simulink model "Beclhoff_Matlab_SimulinkPositionControl"  (R2019a)
settings: Solver=ode3  StartTime=0.0  StopTime=10.0  RelTol=1e-3
libraries: TcTargetLib x7, simulink x1
settings Model: Creator=ChrisK  LastModifiedBy=cknig
settings OptimizationCC: LocalBlockOutputs=off
settings RTWCC: SystemTargetFile=TwinCAT.tlc  GenCodeOnly=on  MakeCommand=make_tct  TemplateMakefile=tct_msbuild.tmf  Description=TwinCAT Target  GenerateReport=on  TargetLang=C++
settings STFCustomTargetCC: TargetLangStandard=C++03 (ISO)  CompOptLevelCompliant=on  MATLABClassNameForMDSCustomization=Simulink.SoftwareTarget.TargetSpecificTriggerConfigurationBase  SystemTargetFile=TwinCAT.tlc

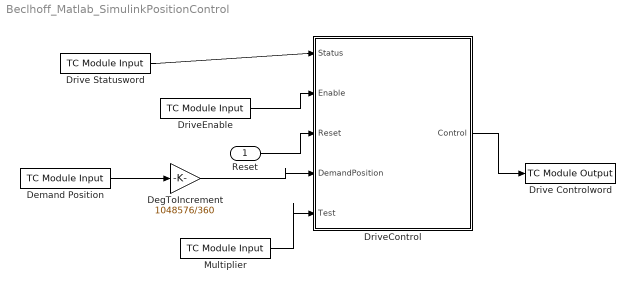
== system Beclhoff_Matlab_SimulinkPositionControl ==
  Reset : Inport  OutDataTypeStr=boolean
  DegToIncrement : Gain  Gain=1048576/360  OutDataTypeStr=int32
  Demand Position : TcTargetLib/TC Module Input  PortDataType=uint8  PortDim=1  Value=0  SampleTime=-1  CodeGenConnectType=DataArea (InputDst)
      settings: SourceProductName=Beckhoff TwinCAT Target
  "Drive Controlword " : TcTargetLib/TC Module Output  PortDataType=uint16  PortDim=1  SampleTime=-1  CodeGenConnectType=DataArea (OutputSrc)
      settings: SourceProductName=Beckhoff TwinCAT Target
  "Drive Statusword " : TcTargetLib/TC Module Input  PortDataType=uint8  PortDim=1  Value=0  SampleTime=-1  CodeGenConnectType=DataArea (InputDst)
      settings: SourceProductName=Beckhoff TwinCAT Target
  DriveControl : Stateflow chart  BlockKeywords=__PRM__SERIALIZED__DATA__:Stateflow Chart,Stateflow Diagram  TreatAsAtomicUnit=on
  DriveEnable : TcTargetLib/TC Module Input  PortDataType=boolean  PortDim=1  Value=0  SampleTime=-1  CodeGenConnectType=DataArea (InputDst)
      settings: SourceProductName=Beckhoff TwinCAT Target
  "Multiplier " : TcTargetLib/TC Module Input  PortDataType=int32  PortDim=1  Value=0  SampleTime=-1  CodeGenConnectType=DataArea (InputDst)
      settings: SourceProductName=Beckhoff TwinCAT Target
  wires:
  "Drive Statusword "/1 -> DriveControl/1(Status)
  DriveControl/1(Control) -> "Drive Controlword "/1
  DriveEnable/1 -> DriveControl/2(Enable)
  Reset/1 -> DriveControl/3(Reset)
  Demand Position/1 -> DegToIncrement/1
  DegToIncrement/1 -> DriveControl/4(DemandPosition)
  "Multiplier "/1 -> DriveControl/5(Test)

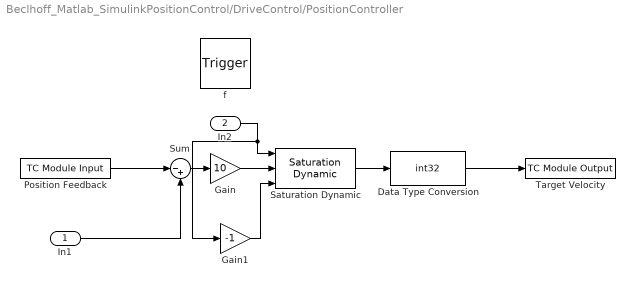
== system Beclhoff_Matlab_SimulinkPositionControl/DriveControl/PositionController ==
  In1 : Inport  OutDataTypeStr=int32  PortDimensions=1
  In2 : Inport  Port=2  OutDataTypeStr=int32  PortDimensions=1
  f : TriggerPort  TriggerType=function-call  VariantControl=(inherit)
      settings: CopyFcn=Stateflow.SLINSF.SimulinkMan.removeBlockPreDeleteFcn  PreDeleteFcn=Stateflow.SLINSF.SimulinkMan.unsafePredeleteFcn
  Data Type Conversion : DataTypeConversion  OutDataTypeStr=int32  SaturateOnIntegerOverflow=on
  Gain : Gain  Gain=10
  Gain1 : Gain  Gain=-1
  "Position Feedback " : TcTargetLib/TC Module Input  PortDataType=int32  PortDim=1  Value=0  SampleTime=-1  CodeGenConnectType=DataArea (InputDst)
      settings: SourceProductName=Beckhoff TwinCAT Target
  Saturation Dynamic : simulink/Discontinuities/Saturation Dynamic  OutMin=[]  OutMax=[]  OutDataTypeStr=Inherit: Same as second input  OutDataType=fixdt(1, 16)  OutScaling=2^-10  DoSatur=off
  Sum : Sum  Inputs=|-+
  Target Velocity : TcTargetLib/TC Module Output  PortDataType=int32  PortDim=1  SampleTime=-1  CodeGenConnectType=DataArea (OutputSrc)
      settings: SourceProductName=Beckhoff TwinCAT Target
  wires:
  Sum/1 -> Gain/1
  "Position Feedback "/1 -> Sum/1
  Data Type Conversion/1 -> Target Velocity/1
  In1/1 -> Sum/2
  Saturation Dynamic/1 -> Data Type Conversion/1
  Gain/1 -> Saturation Dynamic/2
  In2/1 -> Gain1/1, Saturation Dynamic/1
  Gain1/1 -> Saturation Dynamic/3

== stateflow chart Beclhoff_Matlab_SimulinkPositionControl/DriveControl ==
  state NotReady
    entry: Control = 128;
  state SwitchOnDisabled
    entry: Control = 6;
  state WaitForSafety
  state Resetting
    entry: Control = 128;
  state ReadyToSwitchOn
    entry: Control = 7;
  state WaitForEnable
  state Fault
  state SwitchedOn
    entry: Control = 15;
  state PositionController(In1,In2) [function]
  state OperationEnabled
    during: PositionController(DemandPosition,Test);
  (default) -> NotReady
  Resetting -> NotReady : [Status == 96]
  SwitchOnDisabled -> NotReady [order 1] : [Status == 0]
  NotReady -> SwitchOnDisabled : [Status == 96]
  SwitchOnDisabled -> WaitForSafety [order 2] : [Status == 161]
  SwitchOnDisabled -> ReadyToSwitchOn [order 3] : [Status == 33]
  ReadyToSwitchOn -> SwitchOnDisabled [order 1] : [Status == 96]
  WaitForSafety -> ReadyToSwitchOn : [Status == 33]
  SwitchedOn -> ReadyToSwitchOn [order 2] : [Status ==33]
  ReadyToSwitchOn -> WaitForEnable [order 2] : [Status == 35]
  Fault -> Resetting : [Reset == true]
  WaitForEnable -> Fault [order 2] : [Status == 40]
  WaitForEnable -> SwitchedOn [order 1] : [Enable == true]
  OperationEnabled -> Fault [order 2] : [Status == 40]
  SwitchedOn -> Fault [order 3] : [Status ==40]
  SwitchedOn -> OperationEnabled [order 1] : [Status == 39]
  OperationEnabled -> SwitchedOn [order 1] : [Status == 35]
  data: In1 function_input int32 size=1; In2 function_input int32 size=1; Status input; Enable input; Control output uint16; Reset input; DemandPosition input int32; Test input
